simulink library "UAVdesign_net"  (Simulink 7.7)
settings: Solver=ode45  SolverMode=SingleTasking  StartTime=0.0  StopTime=10.0  RelTol=1e-3
undefined symbols (not defined in the file or in its folder): alpha_IERA_IELA_IELA, R_IERA_RA_RA
libraries: UAVdesign_net x75, simulink x13
(part 5 of 8)

== system UAVdesign_net/Utilities/Math/Quaternion Modulus ==
  q : Inport
  Math Function : Math  Operator=sqrt  SaturateOnIntegerOverflow=on
  Quaternion Norm : UAVdesign_net/Utilities/Math/Quaternion Norm  SystemSampleTime=-1
  |q| : Outport
  wires:
  Math Function/1 -> |q|/1
  q/1 -> Quaternion Norm/1
  Quaternion Norm/1 -> Math Function/1

== system UAVdesign_net/Utilities/Math/Quaternion Multiplication ==
  q : Inport
  r : Inport  Port=2
  Mux : Mux
  q0 : Subsystem
  q1 : Subsystem
  q2 : Subsystem
  q3 : Subsystem
  q*r : Outport
  wires:
  q/1 -> q0/1(q), q1/1(q), q2/1(q), q3/1(q)
  r/1 -> q0/2(r), q1/2(r), q2/2(r), q3/2(r)
  q0/1(q0) -> Mux/1
  q1/1(q1) -> Mux/2
  q2/1(q2) -> Mux/3
  q3/1(q3) -> Mux/4
  Mux/1 -> q*r/1

== system UAVdesign_net/Utilities/Math/Quaternion Norm ==
  q : Inport
  Demux : Demux
  Product{,1..3} (4 alike) : Product
  Sum : Sum  Inputs=4
  norm(q) : Outport
  wires:
  q/1 -> Demux/1
  Sum/1 -> norm(q)/1
  Product/1 -> Sum/1
  Product1/1 -> Sum/2
  Product2/1 -> Sum/3
  Product3/1 -> Sum/4
  Demux/1 -> Product/2, Product/1
  Demux/2 -> Product1/2, Product1/1
  Demux/3 -> Product2/2, Product2/1
  Demux/4 -> Product3/2, Product3/1

== system UAVdesign_net/Utilities/Math/Quaternion Normalize ==
  q : Inport
  Demux : Demux
  Mux : Mux
  Product{,1..3} (4 alike) : Product  Inputs=*/
  Quaternion Modulus : UAVdesign_net/Utilities/Math/Quaternion Modulus  SystemSampleTime=-1
  normal(q) : Outport
  wires:
  Demux/4 -> Product3/1
  Demux/3 -> Product2/1
  Demux/2 -> Product1/1
  Demux/1 -> Product/1
  Mux/1 -> normal(q)/1
  q/1 -> Quaternion Modulus/1, Demux/1
  Quaternion Modulus/1 -> Product1/2, Product/2, Product2/2, Product3/2
  Product/1 -> Mux/1
  Product1/1 -> Mux/2
  Product2/1 -> Mux/3
  Product3/1 -> Mux/4

== system UAVdesign_net/Utilities/Math/Quaternion Rotation (B<E) ==
  q : Inport
  v : Inport  Port=2
  Mux : Mux  Inputs=3
  Quaternion Normalize : UAVdesign_net/Utilities/Math/Quaternion Normalize  SystemSampleTime=-1
  V1 : Subsystem
  V2 : Subsystem
  V3 : Subsystem
  q*vq : Outport
  wires:
  Mux/1 -> q*vq/1
  V3/1(V3) -> Mux/3
  V2/1(V2) -> Mux/2
  V1/1(V1) -> Mux/1
  v/1 -> V3/2(vec), V2/2(vec), V1/2(vec)
  q/1 -> Quaternion Normalize/1
  Quaternion Normalize/1 -> V3/1(q), V2/1(q), V1/1(q)

== system UAVdesign_net/Utilities/Math/Quaternion Rotation (E<B) ==
  q : Inport
  v : Inport  Port=2
  Mux : Mux  Inputs=3
  Quaternion Conjugate : UAVdesign_net/Utilities/Math/Quaternion Conjugate  SystemSampleTime=-1
  Quaternion Normalize : UAVdesign_net/Utilities/Math/Quaternion Normalize  SystemSampleTime=-1
  V1 : Subsystem
  V2 : Subsystem
  V3 : Subsystem
  q*vq : Outport
  wires:
  Quaternion Conjugate/1 -> V1/1(q), V2/1(q), V3/1(q)
  Quaternion Normalize/1 -> Quaternion Conjugate/1
  q/1 -> Quaternion Normalize/1
  v/1 -> V1/2(vec), V2/2(vec), V3/2(vec)
  V1/1(V1) -> Mux/1
  V2/1(V2) -> Mux/2
  V3/1(V3) -> Mux/3
  Mux/1 -> q*vq/1

== system UAVdesign_net/Utilities/Math/Quaternion to Vector ==
  q : Inport
  Selector : Selector  InputPortWidth=4  IndexOptions=Index vector (dialog)  Indices=[2 3 4]  OutputSizes=1
  v : Outport
  wires:
  Selector/1 -> v/1
  q/1 -> Selector/1

== system UAVdesign_net/Utilities/Math/SinCos ==
  theta : Inport
  cosine : Trigonometry  Operator=cos
  sine : Trigonometry
  sin(theta) : Outport
  cos(theta) : Outport  Port=2
  wires:
  theta/1 -> sine/1, cosine/1
  sine/1 -> sin(theta)/1
  cosine/1 -> cos(theta)/1

== system UAVdesign_net/Utilities/Math/Transpose ==
  In : Inport
  Permute Dimensions : PermuteDimensions
  Out : Outport
  wires:
  In/1 -> Permute Dimensions/1
  Permute Dimensions/1 -> Out/1

== system UAVdesign_net/Utilities/Math/Vector to Quaternion ==
  v : Inport
  Ground : Ground
  Mux : Mux  Inputs=2
  q : Outport
  wires:
  Ground/1 -> Mux/1
  v/1 -> Mux/2
  Mux/1 -> q/1

== system UAVdesign_net/Utilities/Unit Conversion/Angle Conversion ==
  In1 : Inport
  Unit Conversion : Gain  Gain=slope  SaturateOnIntegerOverflow=on  OutDataTypeStr=Inherit: Same as input  ParamDataTypeStr=Inherit: Same as input
  Out1 : Outport
  wires:
  Unit Conversion/1 -> Out1/1
  In1/1 -> Unit Conversion/1

== system UAVdesign_net/Vehicle Models/Helicopter Model/6 DoF EoM ==
  Environment : Inport  OutDataTypeStr=Bus: Environment
  x : Inport  Port=2
  m : Inport  Port=3
  Inb : Inport  Port=4
  FM_MR : Inport  Port=5
  FM_TR : Inport  Port=6
  FM_FUSE : Inport  Port=7
  FM_HW : Inport  Port=8
  FM_VF : Inport  Port=9
  6DoF Equations of Motion : UAVdesign_net/Equations of Motion/6DoF Equations of Motion  SystemSampleTime=-1
  Add : Sum  Inputs=+++++
  Bus Selector1 : BusSelector  OutputSignals=g
  Constant : Constant  Value=[0 0]
  Constant1 : Constant  Value=[0 0 0 0]
  Constant2 : Constant  Value=[0 0 0 0]
  Constant3 : Constant  Value=[0 0 0]
  Demux : Demux  Outputs=2
  Demux1 : Demux  Outputs=[4 4 3 3 3 3]
  Mux : Mux  Inputs=2
  Mux2 : Mux  Inputs=2
  Product : Product  RndMeth=Zero
  Product1 : Product  Multiplication=Matrix(*)  RndMeth=Zero
  Rotation Matrix from Earth to Body : UAVdesign_net/Utilities/Axes/Euler Rotation Matrix from Earth to Body  SystemSampleTime=-1
  Sum : Sum  Inputs=++|
  Terminator : Terminator
  Terminator1 : Terminator
  Vector Concatenate1 : Concatenate  NumInputs=6  Mode=Vector
  Vector Concatenate6 : Concatenate  NumInputs=6  Mode=Vector
  x_dot : Outport
  FM_CG : Outport  Port=2  PortDimensions=36
  FM_Gravity : Outport  Port=3  PortDimensions=6
  wires:
  Mux2/1 -> FM_Gravity/1, Vector Concatenate6/1  "FM_CG"
  Vector Concatenate6/1 -> FM_CG/1
  Constant3/1 -> Mux2/2
  Vector Concatenate1/1 -> x_dot/1
  6DoF Equations of Motion/4 -> Vector Concatenate1/6  "alpha_E_dot"
  6DoF Equations of Motion/2 -> Vector Concatenate1/5  "omega_B_dot"
  6DoF Equations of Motion/3 -> Vector Concatenate1/4  "R_E_dot"
  6DoF Equations of Motion/1 -> Vector Concatenate1/3  "V_B_dot"
  Constant2/1 -> Vector Concatenate1/2  "p_BE_ddot"
  Constant1/1 -> Vector Concatenate1/1  "p_BE_dot"
  Demux1/1 -> Terminator1/1  "p_BE"
  Demux1/2 -> Terminator/1  "p_BE_dot"
  Demux1/4 -> 6DoF Equations of Motion/3  "R_E"
  Demux1/5 -> 6DoF Equations of Motion/2  "omega_B"
  Demux1/3 -> 6DoF Equations of Motion/1  "V_B"
  Demux1/6 -> Rotation Matrix from Earth to Body/1, 6DoF Equations of Motion/4  "alpha_E"
  Add/1 -> Demux/1
  FM_VF/1 -> Vector Concatenate6/6, Add/5  "FM_VF"
  FM_HW/1 -> Vector Concatenate6/5, Add/4  "FM_HW"
  FM_FUSE/1 -> Vector Concatenate6/4, Add/3  "FM_FUSE"
  FM_TR/1 -> Vector Concatenate6/3, Add/2  "FM_TR"
  FM_MR/1 -> Vector Concatenate6/2, Add/1  "FM_MR"
  Mux/1 -> Product1/2
  Product1/1 -> Mux2/1, Sum/1
  Sum/1 -> 6DoF Equations of Motion/5
  Demux/1 -> Sum/2  "F"
  Rotation Matrix from Earth to Body/1 -> Product1/1
  Product/1 -> Mux/2
  Constant/1 -> Mux/1
  Bus Selector1/1 -> Product/1  "<g>"
  Environment/1 -> Bus Selector1/1
  x/1 -> Demux1/1
  Inb/1 -> 6DoF Equations of Motion/8
  m/1 -> Product/2, 6DoF Equations of Motion/7
  Demux/2 -> 6DoF Equations of Motion/6  "M"

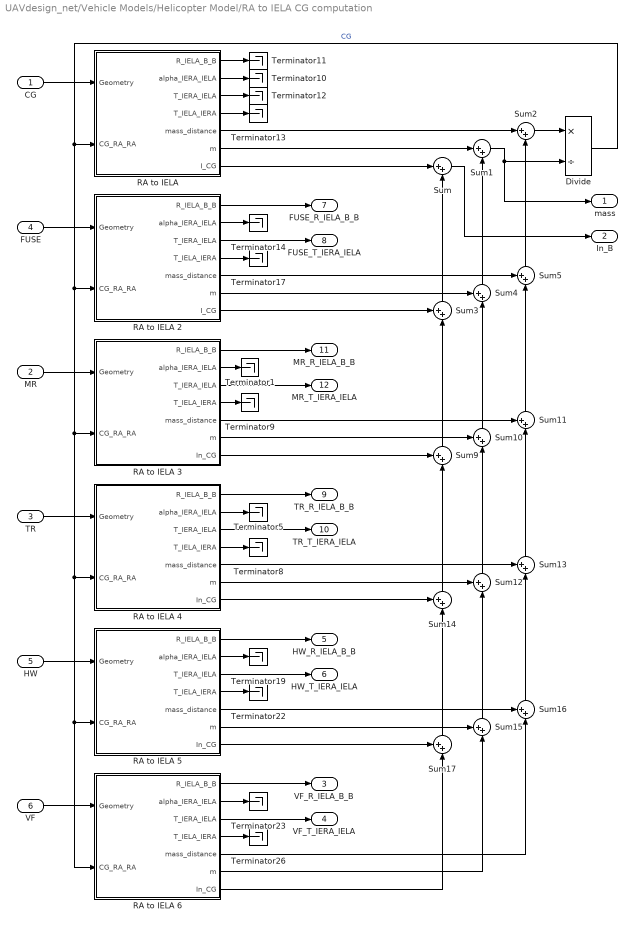
== system UAVdesign_net/Vehicle Models/Helicopter Model/RA to IELA CG computation ==
  CG : Inport  OutDataTypeStr=Bus: GeometryParameters
  MR : Inport  Port=2  OutDataTypeStr=Bus: GeometryParameters
  TR : Inport  Port=3  OutDataTypeStr=Bus: GeometryParameters
  FUSE : Inport  Port=4  OutDataTypeStr=Bus: GeometryParameters
  HW : Inport  Port=5  OutDataTypeStr=Bus: GeometryParameters
  VF : Inport  Port=6  OutDataTypeStr=Bus: GeometryParameters
  Divide : Product  Inputs=*/
  RA to IELA : Subsystem
      mask Display:
      | port_label('input', 1, 'Geometry', 'texmode', 'on')
      | port_label('input', 2, 'R_{CG-RA|RA}', 'texmode', 'on')
      | port_label('output', 1, 'R_{IELA-B|B}', 'texmode', 'on')
      | port_label('output', 2, '\alpha_{IERA-IELA|IELA}', 'texmode', 'on')
      | port_label('output', 3, 'T_{IERA-IELA}', 'texmode', 'on')
      | port_label('output', 4, 'T_{IELA-IERA}', 'texmode', 'on')
      | port_label('output', 5, 'mass x distance', 'texmode', 'on')
      | port_label('output', 6, 'mass', 'texmode', 'on')
      | port_label('output', 7, 'I_{B}', 'texmode', 'on')
  RA to IELA 2 : Subsystem
      mask Display:
      | port_label('input', 1, 'Geometry', 'texmode', 'on')
      | port_label('input', 2, 'R_{CG-RA|RA}', 'texmode', 'on')
      | port_label('output', 1, 'R_{IELA-B|B}', 'texmode', 'on')
      | port_label('output', 2, '\alpha_{IERA-IELA|IELA}', 'texmode', 'on')
      | port_label('output', 3, 'T_{IERA-IELA}', 'texmode', 'on')
      | port_label('output', 4, 'T_{IELA-IERA}', 'texmode', 'on')
      | port_label('output', 5, 'mass x distance', 'texmode', 'on')
      | port_label('output', 6, 'mass', 'texmode', 'on')
      | port_label('output', 7, 'I_{B}', 'texmode', 'on')
  RA to IELA 3 : Subsystem
      mask Display:
      | port_label('input', 1, 'Geometry', 'texmode', 'on')
      | port_label('input', 2, 'R_{CG-RA|RA}', 'texmode', 'on')
      | port_label('output', 1, 'R_{IELA-B|B}', 'texmode', 'on')
      | port_label('output', 2, '\alpha_{IERA-IELA|IELA}', 'texmode', 'on')
      | port_label('output', 3, 'T_{IERA-IELA}', 'texmode', 'on')
      | port_label('output', 4, 'T_{IELA-IERA}', 'texmode', 'on')
      | port_label('output', 5, 'mass x distance', 'texmode', 'on')
      | port_label('output', 6, 'mass', 'texmode', 'on')
      | port_label('output', 7, 'In_{B}', 'texmode', 'on')
  RA to IELA 4 : Subsystem
      mask Display:
      | port_label('input', 1, 'Geometry', 'texmode', 'on')
      | port_label('input', 2, 'R_{CG-RA|RA}', 'texmode', 'on')
      | port_label('output', 1, 'R_{IELA-B|B}', 'texmode', 'on')
      | port_label('output', 2, '\alpha_{IERA-IELA|IELA}', 'texmode', 'on')
      | port_label('output', 3, 'T_{IERA-IELA}', 'texmode', 'on')
      | port_label('output', 4, 'T_{IELA-IERA}', 'texmode', 'on')
      | port_label('output', 5, 'mass x distance', 'texmode', 'on')
      | port_label('output', 6, 'mass', 'texmode', 'on')
      | port_label('output', 7, 'In_{B}', 'texmode', 'on')
  RA to IELA 5 : Subsystem
      mask Display:
      | port_label('input', 1, 'Geometry', 'texmode', 'on')
      | port_label('input', 2, 'R_{CG-RA|RA}', 'texmode', 'on')
      | port_label('output', 1, 'R_{IELA-B|B}', 'texmode', 'on')
      | port_label('output', 2, '\alpha_{IERA-IELA|IELA}', 'texmode', 'on')
      | port_label('output', 3, 'T_{IERA-IELA}', 'texmode', 'on')
      | port_label('output', 4, 'T_{IELA-IERA}', 'texmode', 'on')
      | port_label('output', 5, 'mass x distance', 'texmode', 'on')
      | port_label('output', 6, 'mass', 'texmode', 'on')
      | port_label('output', 7, 'In_{B}', 'texmode', 'on')
  RA to IELA 6 : Subsystem
      mask Display:
      | port_label('input', 1, 'Geometry', 'texmode', 'on')
      | port_label('input', 2, 'R_{CG-RA|RA}', 'texmode', 'on')
      | port_label('output', 1, 'R_{IELA-B|B}', 'texmode', 'on')
      | port_label('output', 2, '\alpha_{IERA-IELA|IELA}', 'texmode', 'on')
      | port_label('output', 3, 'T_{IERA-IELA}', 'texmode', 'on')
      | port_label('output', 4, 'T_{IELA-IERA}', 'texmode', 'on')
      | port_label('output', 5, 'mass x distance', 'texmode', 'on')
      | port_label('output', 6, 'mass', 'texmode', 'on')
      | port_label('output', 7, 'In_{B}', 'texmode', 'on')
  Sum : Sum  Inputs=|++
  Sum1 : Sum  Inputs=|++
  Sum{3..5,9..17} (12 alike) : Sum  Inputs=++|
  Sum2 : Sum  Inputs=|++
  Terminator{1,5,8..14,17,19,22..23,26} (14 alike) : Terminator
  mass : Outport
  In_B : Outport  Port=2
  VF_R_IELA_B_B : Outport  Port=3
  VF_T_IERA_IELA : Outport  Port=4
  HW_R_IELA_B_B : Outport  Port=5
  HW_T_IERA_IELA : Outport  Port=6
  FUSE_R_IELA_B_B : Outport  Port=7
  FUSE_T_IERA_IELA : Outport  Port=8
  TR_R_IELA_B_B : Outport  Port=9
  TR_T_IERA_IELA : Outport  Port=10
  MR_R_IELA_B_B : Outport  Port=11
  MR_T_IERA_IELA : Outport  Port=12
  wires:
  RA to IELA 6/3(T_IERA_IELA) -> VF_T_IERA_IELA/1
  RA to IELA 6/1(R_IELA_B_B) -> VF_R_IELA_B_B/1
  RA to IELA 5/3(T_IERA_IELA) -> HW_T_IERA_IELA/1
  RA to IELA 5/1(R_IELA_B_B) -> HW_R_IELA_B_B/1
  RA to IELA 4/3(T_IERA_IELA) -> TR_T_IERA_IELA/1
  RA to IELA 4/1(R_IELA_B_B) -> TR_R_IELA_B_B/1
  RA to IELA 2/3(T_IERA_IELA) -> FUSE_T_IERA_IELA/1
  RA to IELA 2/1(R_IELA_B_B) -> FUSE_R_IELA_B_B/1
  RA to IELA 6/6(m) -> Sum15/2
  RA to IELA 6/5(mass_distance) -> Sum16/2
  RA to IELA 6/7(In_CG) -> Sum17/2
  RA to IELA 6/4(T_IELA_IERA) -> Terminator26/1
  RA to IELA 6/2(alpha_IERA_IELA) -> Terminator23/1
  VF/1 -> RA to IELA 6/1(Geometry)
  RA to IELA 5/6(m) -> Sum15/1
  RA to IELA 5/5(mass_distance) -> Sum16/1
  Sum16/1 -> Sum13/2
  Sum15/1 -> Sum12/2
  Sum17/1 -> Sum14/2
  RA to IELA 5/7(In_CG) -> Sum17/1
  RA to IELA 5/4(T_IELA_IERA) -> Terminator22/1
  RA to IELA 5/2(alpha_IERA_IELA) -> Terminator19/1
  HW/1 -> RA to IELA 5/1(Geometry)
  RA to IELA 4/6(m) -> Sum12/1
  RA to IELA 4/5(mass_distance) -> Sum13/1
  Sum13/1 -> Sum11/2
  Sum12/1 -> Sum10/2
  Sum14/1 -> Sum9/2
  RA to IELA 4/7(In_CG) -> Sum14/1
  RA to IELA 3/5(mass_distance) -> Sum11/1
  RA to IELA 3/6(m) -> Sum10/1
  Sum11/1 -> Sum5/2
  Sum10/1 -> Sum4/2
  Sum9/1 -> Sum3/2
  RA to IELA 3/7(In_CG) -> Sum9/1
  FUSE/1 -> RA to IELA 2/1(Geometry)
  Sum2/1 -> Divide/1
  Sum1/1 -> mass/1, Divide/2
  Sum/1 -> In_B/1
  Sum5/1 -> Sum2/2
  Sum4/1 -> Sum1/2
  Sum3/1 -> Sum/2
  RA to IELA 2/7(I_CG) -> Sum3/1
  RA to IELA 2/5(mass_distance) -> Sum5/1
  RA to IELA 2/6(m) -> Sum4/1
  RA to IELA 2/4(T_IELA_IERA) -> Terminator17/1
  RA to IELA 2/2(alpha_IERA_IELA) -> Terminator14/1
  RA to IELA/5(mass_distance) -> Sum2/1
  RA to IELA/6(m) -> Sum1/1
  RA to IELA/7(I_CG) -> Sum/1
  RA to IELA/4(T_IELA_IERA) -> Terminator13/1
  RA to IELA/3(T_IERA_IELA) -> Terminator12/1
  RA to IELA/1(R_IELA_B_B) -> Terminator11/1
  RA to IELA/2(alpha_IERA_IELA) -> Terminator10/1
  CG/1 -> RA to IELA/1(Geometry)
  Divide/1 -> RA to IELA 3/2(CG_RA_RA), RA to IELA 4/2(CG_RA_RA), RA to IELA 5/2(CG_RA_RA), RA to IELA 6/2(CG_RA_RA), RA to IELA 2/2(CG_RA_RA), RA to IELA/2(CG_RA_RA)  "CG"
  RA to IELA 3/4(T_IELA_IERA) -> Terminator9/1
  RA to IELA 4/4(T_IELA_IERA) -> Terminator8/1
  RA to IELA 4/2(alpha_IERA_IELA) -> Terminator5/1
  TR/1 -> RA to IELA 4/1(Geometry)
  RA to IELA 3/3(T_IERA_IELA) -> MR_T_IERA_IELA/1
  RA to IELA 3/2(alpha_IERA_IELA) -> Terminator1/1
  RA to IELA 3/1(R_IELA_B_B) -> MR_R_IELA_B_B/1
  MR/1 -> RA to IELA 3/1(Geometry)

== system UAVdesign_net/Vehicle Models/Helicopter Model/Wash Coupling ==
  d_vector : Inport
  ParametersBus : Inport  Port=2
  GeometryBus : Inport  Port=3
  Bus Selector : BusSelector  OutputSignals=MR.radius
  Bus Selector1 : BusSelector  OutputSignals=MR.R_IERA_RA_RA,TR.R_IERA_RA_RA,FUSE.R_IERA_RA_RA,HW.R_IERA_RA_RA,VF.R_IERA_RA_RA
  Vector Concatenate1 : Concatenate  NumInputs=5  Mode=Vector
  Wash Coupling : Stateflow chart  TreatAsAtomicUnit=on
  V_W_omega_W_vector : Outport
  wires:
  Bus Selector1/5 -> Vector Concatenate1/5  "<R_IERA_RA_RA>"
  Bus Selector1/4 -> Vector Concatenate1/4  "<R_IERA_RA_RA>"
  Bus Selector1/3 -> Vector Concatenate1/3  "<R_IERA_RA_RA>"
  Bus Selector1/2 -> Vector Concatenate1/2  "<R_IERA_RA_RA>"
  Bus Selector1/1 -> Vector Concatenate1/1  "<R_IERA_RA_RA>"
  Vector Concatenate1/1 -> Wash Coupling/2(R)
  GeometryBus/1 -> Bus Selector1/1
  Bus Selector/1 -> Wash Coupling/3(MR_radius)  "<radius>"
  ParametersBus/1 -> Bus Selector/1
  Wash Coupling/1(vw_omw) -> V_W_omega_W_vector/1
  d_vector/1 -> Wash Coupling/1(d)

== system UAVdesign_net/Vehicle Models/Helicopter Parameters/Fin Parameters ==
  In : Inport
  Bus Creator : BusCreator  Inputs=14  OutDataTypeStr=Bus: FinParameters  NonVirtualBus=on
  Demux : Demux  Outputs=14
  Gain{,1..3} (4 alike) : Gain  Gain=pi/180
  Parameters : Outport  OutDataTypeStr=Bus: FinParameters
  wires:
  In/1 -> Demux/1
  Bus Creator/1 -> Parameters/1
  Demux/1 -> Bus Creator/1  "span"
  Demux/2 -> Bus Creator/2  "chord"
  Demux/3 -> Gain2/1
  Gain2/1 -> Bus Creator/3  "dihedral"
  Demux/4 -> Gain/1
  Gain/1 -> Bus Creator/4  "incid"
  Gain1/1 -> Bus Creator/5  "sweep"
  Demux/5 -> Gain1/1
  Demux/6 -> Bus Creator/6  "taper"
  Demux/7 -> Gain3/1
  Gain3/1 -> Bus Creator/7  "stall"
  Demux/8 -> Bus Creator/8  "a0"
  Demux/9 -> Bus Creator/9  "a1s2"
  Demux/10 -> Bus Creator/10  "cd0"
  Demux/11 -> Bus Creator/11  "cd1s1"
  Demux/12 -> Bus Creator/12  "cd2c1"
  Demux/13 -> Bus Creator/13  "cm0"
  Demux/14 -> Bus Creator/14  "cm1s1"

== system UAVdesign_net/Vehicle Models/Helicopter Parameters/Fin Parameters1 ==
  In : Inport
  Bus Creator : BusCreator  Inputs=14  OutDataTypeStr=Bus: FinParameters  NonVirtualBus=on
  Demux : Demux  Outputs=14
  Gain{,1..3} (4 alike) : Gain  Gain=pi/180
  Parameters : Outport  OutDataTypeStr=Bus: FinParameters
  wires:
  Demux/14 -> Bus Creator/14  "cm1s1"
  Demux/13 -> Bus Creator/13  "cm0"
  Demux/12 -> Bus Creator/12  "cd2c1"
  Demux/11 -> Bus Creator/11  "cd1s1"
  Demux/10 -> Bus Creator/10  "cd0"
  Demux/9 -> Bus Creator/9  "a1s2"
  Demux/8 -> Bus Creator/8  "a0"
  Gain3/1 -> Bus Creator/7  "stall"
  Demux/7 -> Gain3/1
  Demux/6 -> Bus Creator/6  "taper"
  Demux/5 -> Gain1/1
  Gain1/1 -> Bus Creator/5  "sweep"
  Gain/1 -> Bus Creator/4  "incid"
  Demux/4 -> Gain/1
  Gain2/1 -> Bus Creator/3  "dihedral"
  Demux/3 -> Gain2/1
  Demux/2 -> Bus Creator/2  "chord"
  Demux/1 -> Bus Creator/1  "span"
  Bus Creator/1 -> Parameters/1
  In/1 -> Demux/1

== system UAVdesign_net/Vehicle Models/Helicopter Parameters/Fuse Parameters ==
  In : Inport
  Bus Creator : BusCreator  Inputs=7  OutDataTypeStr=Bus: FuselageParameters  NonVirtualBus=on
  Demux : Demux  Outputs=17
  Vector Concatenate{,1..4} (5 alike) : Concatenate  NumInputs=3  Mode=Vector
  Parameters : Outport  OutDataTypeStr=Bus: FuselageParameters
  wires:
  Demux/1 -> Bus Creator/1  "carea"
  Bus Creator/1 -> Parameters/1
  In/1 -> Demux/1
  Demux/2 -> Bus Creator/2  "clen"
  Demux/3 -> Vector Concatenate/1
  Demux/4 -> Vector Concatenate/2
  Demux/5 -> Vector Concatenate/3
  Vector Concatenate/1 -> Bus Creator/3  "cx"
  Demux/6 -> Vector Concatenate1/1
  Demux/7 -> Vector Concatenate1/2
  Demux/8 -> Vector Concatenate1/3
  Vector Concatenate1/1 -> Bus Creator/4  "cy"
  Demux/9 -> Vector Concatenate2/1
  Demux/10 -> Vector Concatenate2/2
  Demux/11 -> Vector Concatenate2/3
  Vector Concatenate2/1 -> Bus Creator/5  "cz"
  Demux/12 -> Vector Concatenate3/1
  Demux/13 -> Vector Concatenate3/2
  Demux/14 -> Vector Concatenate3/3
  Demux/15 -> Vector Concatenate4/1
  Demux/16 -> Vector Concatenate4/2
  Demux/17 -> Vector Concatenate4/3
  Vector Concatenate3/1 -> Bus Creator/6  "cm"
  Vector Concatenate4/1 -> Bus Creator/7  "cn"

== system UAVdesign_net/Vehicle Models/Helicopter Parameters/Rotor Parameters ==
  In : Inport
  Bus Creator : BusCreator  Inputs=18  OutDataTypeStr=Bus: RotorParameters  NonVirtualBus=on
  Data Type Conversion : DataTypeConversion  OutDataTypeStr=int32  RndMeth=Nearest
  Data Type Conversion1 : DataTypeConversion  OutDataTypeStr=uint32  RndMeth=Nearest
  Demux : Demux  Outputs=20
  Gain : Gain  Gain=pi/180
  Gain1 : Gain  Gain=pi/180
  Gain2 : Gain  Gain=180/pi
  Gain3 : Gain  Gain=pi/180
  Vector Concatenate : Concatenate  NumInputs=3  Mode=Vector
  Parameters : Outport  OutDataTypeStr=Bus: RotorParameters
  wires:
  Demux/20 -> Bus Creator/18  "azsign"
  Demux/18 -> Bus Creator/16  "lmast"
  Demux/17 -> Bus Creator/15  "mbar"
  Demux/16 -> Bus Creator/14  "iflap"
  Demux/13 -> Bus Creator/11  "btmax"
  Demux/1 -> Bus Creator/1  "a0"
  Bus Creator/1 -> Parameters/1
  Demux/4 -> Vector Concatenate/3
  Demux/3 -> Vector Concatenate/2
  Demux/2 -> Vector Concatenate/1
  Vector Concatenate/1 -> Bus Creator/2  "del0_2"
  In/1 -> Demux/1
  Data Type Conversion/1 -> Bus Creator/17  "hubtype"
  Demux/19 -> Data Type Conversion/1
  Gain/1 -> Bus Creator/3  "precone"
  Gain1/1 -> Bus Creator/4  "delta3"
  Gain2/1 -> Bus Creator/6  "khub"
  Gain3/1 -> Bus Creator/13  "twist"
  Demux/5 -> Gain/1
  Demux/6 -> Gain1/1
  Demux/7 -> Bus Creator/5  "e"
  Demux/8 -> Gain2/1
  Data Type Conversion1/1 -> Bus Creator/7  "nb"
  Demux/9 -> Data Type Conversion1/1
  Demux/10 -> Bus Creator/8  "radius"
  Demux/11 -> Bus Creator/9  "chord"
  Demux/12 -> Bus Creator/10  "btmin"
  Demux/15 -> Gain3/1
  Demux/14 -> Bus Creator/12  "btq"

== system UAVdesign_net/Vehicle Models/Helicopter Parameters/Rotor Parameters1 ==
  In : Inport
  Bus Creator : BusCreator  Inputs=18  OutDataTypeStr=Bus: RotorParameters  NonVirtualBus=on
  Data Type Conversion : DataTypeConversion  OutDataTypeStr=int32  RndMeth=Nearest
  Data Type Conversion1 : DataTypeConversion  OutDataTypeStr=uint32  RndMeth=Nearest
  Demux : Demux  Outputs=20
  Gain : Gain  Gain=pi/180
  Gain1 : Gain  Gain=pi/180
  Gain2 : Gain  Gain=180/pi
  Gain3 : Gain  Gain=pi/180
  Vector Concatenate : Concatenate  NumInputs=3  Mode=Vector
  Parameters : Outport  OutDataTypeStr=Bus: RotorParameters
  wires:
  Demux/14 -> Bus Creator/12  "btq"
  Demux/15 -> Gain3/1
  Demux/12 -> Bus Creator/10  "btmin"
  Demux/11 -> Bus Creator/9  "chord"
  Demux/10 -> Bus Creator/8  "radius"
  Demux/9 -> Data Type Conversion1/1
  Data Type Conversion1/1 -> Bus Creator/7  "nb"
  Demux/8 -> Gain2/1
  Demux/7 -> Bus Creator/5  "e"
  Demux/6 -> Gain1/1
  Demux/5 -> Gain/1
  Gain3/1 -> Bus Creator/13  "twist"
  Gain2/1 -> Bus Creator/6  "khub"
  Gain1/1 -> Bus Creator/4  "delta3"
  Gain/1 -> Bus Creator/3  "precone"
  Demux/19 -> Data Type Conversion/1
  Data Type Conversion/1 -> Bus Creator/17  "hubtype"
  In/1 -> Demux/1
  Vector Concatenate/1 -> Bus Creator/2  "del0_2"
  Demux/2 -> Vector Concatenate/1
  Demux/3 -> Vector Concatenate/2
  Demux/4 -> Vector Concatenate/3
  Bus Creator/1 -> Parameters/1
  Demux/1 -> Bus Creator/1  "a0"
  Demux/13 -> Bus Creator/11  "btmax"
  Demux/16 -> Bus Creator/14  "iflap"
  Demux/17 -> Bus Creator/15  "mbar"
  Demux/18 -> Bus Creator/16  "lmast"
  Demux/20 -> Bus Creator/18  "azsign"

== system UAVdesign_net/Vehicle Models/Quad-Rotor Model (Momentum)/6 DoF EoM ==
  Environment : Inport
  x : Inport  Port=2
  m : Inport  Port=3
  Inb : Inport  Port=4
  FM_ROT : Inport  Port=5
  FM_FUSE : Inport  Port=6
  6DoF Equations of Motion (Quaternions) : UAVdesign_net/Equations of Motion/6DoF Equations of Motion (Quaternions)  SystemSampleTime=-1
  Add : Sum  Inputs=+++++
  Bus Selector1 : BusSelector  OutputSignals=g
  Constant : Constant  Value=[0 0]
  Constant3 : Constant  Value=[0 0 0]
  Demux : Demux  Outputs=2
  Demux1 : Demux  Outputs=[3 3 3 4]
  Demux2 : Demux
  Mux : Mux  Inputs=2
  Mux2 : Mux  Inputs=2
  Product : Product  RndMeth=Zero
  Quaternion Rotation (B<E) : UAVdesign_net/Utilities/Math/Quaternion Rotation (B<E)  SystemSampleTime=-1
  Sum : Sum  Inputs=++|
  Vector Concatenate1 : Concatenate  NumInputs=4  Mode=Vector
  Vector Concatenate6 : Concatenate  NumInputs=3  Mode=Vector
  x_dot : Outport
  FM_CG : Outport  Port=2  PortDimensions=36
  FM_Gravity : Outport  Port=3  PortDimensions=6
  wires:
  Demux/2 -> 6DoF Equations of Motion (Quaternions)/6  "M"
  m/1 -> Product/2, 6DoF Equations of Motion (Quaternions)/7
  Inb/1 -> 6DoF Equations of Motion (Quaternions)/8
  x/1 -> Demux1/1
  Environment/1 -> Bus Selector1/1
  Bus Selector1/1 -> Product/1  "<g>"
  Constant/1 -> Mux/1
  Product/1 -> Mux/2
  Demux/1 -> Sum/2  "F"
  Sum/1 -> 6DoF Equations of Motion (Quaternions)/5
  Add/1 -> Demux/1
  Vector Concatenate1/1 -> x_dot/1
  Constant3/1 -> Mux2/2
  Vector Concatenate6/1 -> FM_CG/1
  FM_FUSE/1 -> Vector Concatenate6/3, Add/5  "FM_FUSE"
  FM_ROT/1 -> Vector Concatenate6/2, Demux2/1  "FM_ROT"
  Mux2/1 -> Vector Concatenate6/1, FM_Gravity/1  "FM_CG"
  Mux/1 -> Quaternion Rotation (B<E)/2
  Demux1/1 -> 6DoF Equations of Motion (Quaternions)/1
  Demux1/2 -> 6DoF Equations of Motion (Quaternions)/2
  Demux1/3 -> 6DoF Equations of Motion (Quaternions)/3
  Demux1/4 -> 6DoF Equations of Motion (Quaternions)/4, Quaternion Rotation (B<E)/1
  Quaternion Rotation (B<E)/1 -> Sum/1, Mux2/1
  6DoF Equations of Motion (Quaternions)/1 -> Vector Concatenate1/1
  6DoF Equations of Motion (Quaternions)/2 -> Vector Concatenate1/2
  6DoF Equations of Motion (Quaternions)/3 -> Vector Concatenate1/3
  6DoF Equations of Motion (Quaternions)/4 -> Vector Concatenate1/4
  Demux2/1 -> Add/1
  Demux2/2 -> Add/2
  Demux2/3 -> Add/3
  Demux2/4 -> Add/4

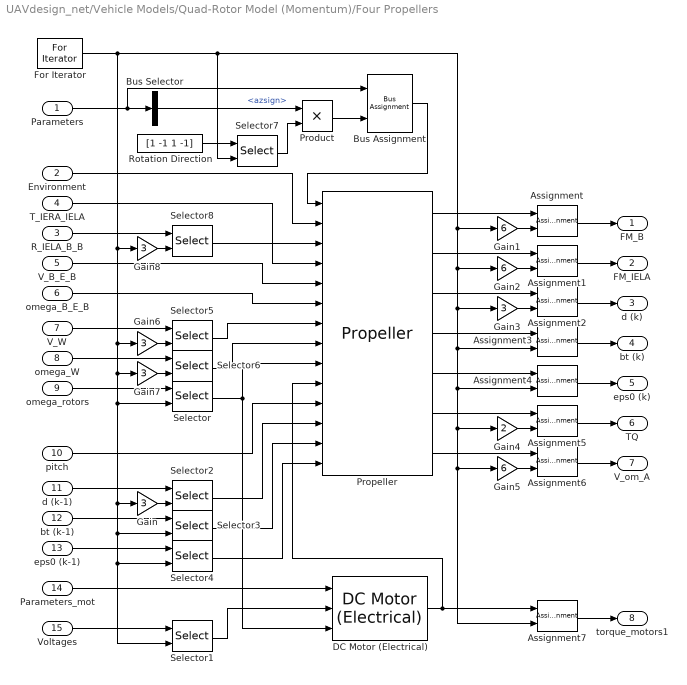
== system UAVdesign_net/Vehicle Models/Quad-Rotor Model (Momentum)/Four Propellers ==
  Parameters : Inport
  Environment : Inport  Port=2
  R_IELA_B_B : Inport  Port=3  PortDimensions=12
  T_IERA_IELA : Inport  Port=4  PortDimensions=[3 3]
  V_B_E_B : Inport  Port=5  PortDimensions=3
  omega_B_E_B : Inport  Port=6  PortDimensions=3
  V_W : Inport  Port=7  PortDimensions=12
  omega_W : Inport  Port=8  PortDimensions=12
  omega_rotors : Inport  Port=9  PortDimensions=4
  pitch : Inport  Port=10  PortDimensions=1
  d (k-1) : Inport  Port=11  PortDimensions=12
  bt (k-1) : Inport  Port=12  PortDimensions=4
  eps0 (k-1) : Inport  Port=13  PortDimensions=4
  Parameters_mot : Inport  Port=14
  Voltages : Inport  Port=15  PortDimensions=4
  Assignment : Assignment  IndexMode=Zero-based  OutputInitialize=Specify size for each dimension in table  IndexOptions=Starting index (port)  Indices=1  OutputSizes=24
  Assignment1 : Assignment  IndexMode=Zero-based  OutputInitialize=Specify size for each dimension in table  IndexOptions=Starting index (port)  Indices=1  OutputSizes=24
  Assignment2 : Assignment  IndexMode=Zero-based  OutputInitialize=Specify size for each dimension in table  IndexOptions=Starting index (port)  Indices=1  OutputSizes=12
  Assignment3 : Assignment  IndexMode=Zero-based  OutputInitialize=Specify size for each dimension in table  IndexOptions=Starting index (port)  Indices=1  OutputSizes=4
  Assignment4 : Assignment  IndexMode=Zero-based  OutputInitialize=Specify size for each dimension in table  IndexOptions=Starting index (port)  Indices=1  OutputSizes=4
  Assignment5 : Assignment  IndexMode=Zero-based  OutputInitialize=Specify size for each dimension in table  IndexOptions=Starting index (port)  Indices=1  OutputSizes=8
  Assignment6 : Assignment  IndexMode=Zero-based  OutputInitialize=Specify size for each dimension in table  IndexOptions=Starting index (port)  Indices=1  OutputSizes=24
  Assignment7 : Assignment  IndexMode=Zero-based  OutputInitialize=Specify size for each dimension in table  IndexOptions=Starting index (port)  Indices=1  OutputSizes=4
  Bus Selector : BusSelector  OutputSignals=azsign
  Bus Assignment : BusAssignment  AssignedSignals=azsign
  DC Motor (Electrical) : UAVdesign_net/Subsystem Models/DC Motor (Electrical)  SystemSampleTime=-1
  For Iterator : ForIterator  ResetStates=reset  IterationLimit=4  IndexMode=Zero-based
  Gain{,3,6..8} (5 alike) : Gain  Gain=3  OutDataTypeStr=uint32
  Gain1 : Gain  Gain=6  OutDataTypeStr=uint32
  Gain2 : Gain  Gain=6  OutDataTypeStr=uint32
  Gain4 : Gain  Gain=2  OutDataTypeStr=uint32
  Gain5 : Gain  Gain=6  OutDataTypeStr=uint32
  Product : Product  RndMeth=Zero
  Propeller : UAVdesign_net/Subsystem Models/Propeller  SystemSampleTime=-1
  Rotation Direction : Constant  Value=[1 -1 1 -1]
  Selector{,1,3..4,7} (5 alike) : Selector  IndexMode=Zero-based  InputPortWidth=4  IndexOptions=Starting index (port)  Indices=[1 3]  OutputSizes=1
  Selector{2,5..6,8} (4 alike) : Selector  IndexMode=Zero-based  InputPortWidth=12  IndexOptions=Starting index (port)  Indices=[1 3]  OutputSizes=3
  FM_B : Outport
  FM_IELA : Outport  Port=2
  d (k) : Outport  Port=3
  bt (k) : Outport  Port=4
  eps0 (k) : Outport  Port=5
  TQ : Outport  Port=6
  V_om_A : Outport  Port=7
  torque_motors1 : Outport  Port=8
  wires:
  Voltages/1 -> Selector1/1
  Selector1/1 -> DC Motor (Electrical)/2
  Assignment7/1 -> torque_motors1/1
  DC Motor (Electrical)/1 -> Propeller/10, Assignment7/1
  Parameters_mot/1 -> DC Motor (Electrical)/1
  Selector4/1 -> Propeller/14
  Selector3/1 -> Propeller/13
  Selector2/1 -> Propeller/12
  pitch/1 -> Propeller/11
  Selector/1 -> DC Motor (Electrical)/3, Propeller/9
  Selector6/1 -> Propeller/8
  Selector5/1 -> Propeller/7
  Gain8/1 -> Selector8/2
  R_IELA_B_B/1 -> Selector8/1
  Selector8/1 -> Propeller/3
  Rotation Direction/1 -> Selector7/1
  Selector7/1 -> Product/2
  Product/1 -> Bus Assignment/2
  Bus Selector/1 -> Product/1  "<azsign>"
  Parameters/1 -> Bus Selector/1, Bus Assignment/1
  Bus Assignment/1 -> Propeller/1
  Gain7/1 -> Selector6/2
  Gain6/1 -> Selector5/2
  omega_W/1 -> Selector6/1
  V_W/1 -> Selector5/1
  Assignment6/1 -> V_om_A/1
  Propeller/7 -> Assignment6/1
  Gain5/1 -> Assignment6/2
  Assignment5/1 -> TQ/1
  Assignment4/1 -> eps0 (k)/1
  Assignment3/1 -> bt (k)/1
  Propeller/6 -> Assignment5/1
  Gain4/1 -> Assignment5/2
  Propeller/5 -> Assignment4/1
  Propeller/4 -> Assignment3/1
  Assignment2/1 -> d (k)/1
  Propeller/3 -> Assignment2/1
  Gain3/1 -> Assignment2/2
  Assignment1/1 -> FM_IELA/1
  Propeller/2 -> Assignment1/1
  Gain2/1 -> Assignment1/2
  Propeller/1 -> Assignment/1
  Gain1/1 -> Assignment/2
  Assignment/1 -> FM_B/1
  eps0 (k-1)/1 -> Selector4/1
  bt (k-1)/1 -> Selector3/1
  d (k-1)/1 -> Selector2/1
  Gain/1 -> Selector2/2
  For Iterator/1 -> Gain8/1, Gain6/1, Gain7/1, Gain/1, Selector1/2, Selector4/2, Selector3/2, Selector/2, Selector7/2, Assignment7/2, Gain5/1, Gain4/1, Assignment4/2, Assignment3/2, Gain3/1, Gain2/1, Gain1/1
  omega_rotors/1 -> Selector/1
  omega_B_E_B/1 -> Propeller/6
  V_B_E_B/1 -> Propeller/5
  T_IERA_IELA/1 -> Propeller/4
  Environment/1 -> Propeller/2

== system UAVdesign_net/Vehicle Models/Quad-Rotor Model (Momentum)/Four Propellers Rotation Dynamics ==
  Parameters : Inport
  torque_prop : Inport  Port=2  PortDimensions=4
  torque_mot : Inport  Port=3  PortDimensions=4
  omega_B_E_B : Inport  Port=4  PortDimensions=3
  omega_dot_B_E_B : Inport  Port=5  PortDimensions=3
  omega_rotors : Inport  Port=6  PortDimensions=4
  Assignment1 : Assignment  IndexMode=Zero-based  OutputInitialize=Specify size for each dimension in table  IndexOptions=Starting index (port)  Indices=1  OutputSizes=4
  Bus Selector : BusSelector  OutputSignals=azsign
  Bus Assignment : BusAssignment  AssignedSignals=azsign
  For Iterator : ForIterator  ResetStates=reset  IterationLimit=4  IndexMode=Zero-based
  Orientation : Constant  Value=eye(3,3)
  Product : Product  RndMeth=Zero
  Propeller Rotation Dynamics : UAVdesign_net/Subsystem Models/Propeller Rotation Dynamics  SystemSampleTime=-1
  Rotation Direction : Constant  Value=[1 -1 1 -1]
  Selector{1..3,7} (4 alike) : Selector  IndexMode=Zero-based  InputPortWidth=4  IndexOptions=Starting index (port)  Indices=[1 3]  OutputSizes=1
  omega_dot_motors : Outport
  wires:
  torque_mot/1 -> Selector3/1
  Selector3/1 -> Propeller Rotation Dynamics/4
  omega_rotors/1 -> Selector2/1
  Rotation Direction/1 -> Selector7/1
  Selector7/1 -> Product/2
  Product/1 -> Bus Assignment/2
  Bus Selector/1 -> Product/1  "<azsign>"
  Parameters/1 -> Bus Selector/1, Bus Assignment/1
  Bus Assignment/1 -> Propeller Rotation Dynamics/1
  For Iterator/1 -> Selector3/2, Selector2/2, Selector1/2, Assignment1/2, Selector7/2
  Orientation/1 -> Propeller Rotation Dynamics/2
  omega_B_E_B/1 -> Propeller Rotation Dynamics/5
  torque_prop/1 -> Selector1/1
  Selector1/1 -> Propeller Rotation Dynamics/3
  omega_dot_B_E_B/1 -> Propeller Rotation Dynamics/6
  Selector2/1 -> Propeller Rotation Dynamics/7
  Assignment1/1 -> omega_dot_motors/1
  Propeller Rotation Dynamics/1 -> Assignment1/1

== system UAVdesign_net/Vehicle Models/Quad-Rotor Model (Momentum)/Fuselage ==
  Parameters : Inport
  Environment : Inport  Port=2
  R_IELA_B_B : Inport  Port=3  PortDimensions=3
  T_IERA_IELA : Inport  Port=4  PortDimensions=[3 3]
  V_B_E_B : Inport  Port=5  PortDimensions=3
  omega_B_E_B : Inport  Port=6  PortDimensions=3
  V_W : Inport  Port=7  PortDimensions=3
  omega_W : Inport  Port=8  PortDimensions=3
  CG to IELA : Subsystem
      mask Display:
      | port_label('input', 1, 'R_{IELA-B|B}', 'texmode', 'on')
      | port_label('input', 2, 'V_{B-E|B}', 'texmode', 'on')
      | port_label('input', 3, '\omega_{B-E|B}', 'texmode', 'on')
      | port_label('output', 1, 'V_{IELA-E|IELA}', 'texmode', 'on')
      | port_label('output', 2, '\omega_{IELA-E|IELA}', 'texmode', 'on')
  Fuselage Model (IERA) : Subsystem
      mask Display:
      | port_label('input', 1, 'Parameters', 'texmode', 'on')
      | port_label('input', 2, 'Environment', 'texmode', 'on')
      | port_label('input', 3, 'V_{A}', 'texmode', 'on')
      | port_label('input', 4, '\omega_{A}', 'texmode', 'on')
      | port_label('input', 5, 'V_{W}', 'texmode', 'on')
      | port_label('input', 6, '\omega_{W}', 'texmode', 'on')
      | 
      | port_label('output', 1, 'FM_{I}', 'texmode', 'on')
      | port_label('output', 2, 'FM_{A}', 'texmode', 'on')
      | port_label('output', 3, 'd_{k}', 'texmode', 'on')
  IELA to CG : Subsystem
      mask Display:
      | port_label('input', 1, 'R_{IELA-B|B}', 'texmode', 'on')
      | port_label('input', 2, 'FM_{IELA}', 'texmode', 'on')
      | port_label('output', 1, 'FM_{B}', 'texmode', 'on')
  IELA to IERA : Subsystem
      mask Display:
      | port_label('input', 1, 'T_{IERA-IELA}', 'texmode', 'on')
      | port_label('input', 2, 'V_{A|IELA}', 'texmode', 'on')
      | port_label('input', 3, '\omega_{A|IELA}', 'texmode', 'on')
      | port_label('input', 4, 'V_{W|IELA}', 'texmode', 'on')
      | port_label('input', 5, '\omega_{W|IELA}', 'texmode', 'on')
      | 
      | port_label('output', 1, 'V_{A|IERA}', 'texmode', 'on')
      | port_label('output', 2, '\omega_{A|IERA}', 'texmode', 'on')
      | port_label('output', 3, 'V_{W|IERA}', 'texmode', 'on')
      | port_label('output', 4, '\omega_{W|IERA}', 'texmode', 'on')
  IERA to IELA : Subsystem
      mask Display:
      | port_label('input', 1, 'T_{IELA-IERA}', 'texmode', 'on')
      | port_label('input', 2, 'FM_{I|IERA}', 'texmode', 'on')
      | port_label('input', 3, 'FM_{A|IERA}', 'texmode', 'on')
      | port_label('input', 4, 'd_{IERA}', 'texmode', 'on')
      | port_label('output', 1, 'FM_{I|IELA}', 'texmode', 'on')
      | port_label('output', 2, 'FM_{A|IELA}', 'texmode', 'on')
      | port_label('output', 3, 'd_{IELA}', 'texmode', 'on')
  Sum : Sum  Inputs=++|
  Sum3 : Sum  Inputs=|+-
  Sum4 : Sum  Inputs=|+-
  Transpose : Subsystem
      mask Display: disp('A^T', 'texmode', 'on')
  Vector Concatenate : Concatenate  Mode=Vector
  FM_B : Outport  PortDimensions=6
  FM_IELA : Outport  Port=2  PortDimensions=6
  d (k) : Outport  Port=3  PortDimensions=3
  V_om_A : Outport  Port=4  PortDimensions=6
  wires:
  Vector Concatenate/1 -> V_om_A/1
  omega_W/1 -> IELA to IERA/5(omega_W_IELA), Sum4/2
  V_W/1 -> IELA to IERA/4(V_W_IELA), Sum3/2
  Sum4/1 -> Vector Concatenate/2, IELA to IERA/3(omega_A_IELA)
  CG to IELA/2(omega_IELA-E|IELA) -> Sum4/1
  Sum3/1 -> Vector Concatenate/1, IELA to IERA/2(V_A_IELA)
  CG to IELA/1(V_IELA-E|IELA) -> Sum3/1
  R_IELA_B_B/1 -> IELA to CG/1(R_IELA_B_B), CG to IELA/1(R_IELA-B|B)
  IERA to IELA/3(d_IELA) -> d (k)/1
  IELA to CG/1(FM_B) -> FM_B/1
  Transpose/1(Out) -> IERA to IELA/1(T_IELA_IERA)
  V_B_E_B/1 -> CG to IELA/2(V_B-E|B)
  T_IERA_IELA/1 -> Transpose/1(In), IELA to IERA/1(T_IERA_IELA)
  Environment/1 -> Fuselage Model (IERA)/2(Environment)
  Parameters/1 -> Fuselage Model (IERA)/1(Parameters)
  Fuselage Model (IERA)/3(d (k)) -> IERA to IELA/4(d_IERA)
  IERA to IELA/2(FM_A_IELA) -> Sum/2
  IELA to IERA/4(omega_W_IERA) -> Fuselage Model (IERA)/6(omega_W)
  IELA to IERA/3(V_W_IERA) -> Fuselage Model (IERA)/5(V_W)
  IELA to IERA/2(omega_A_IERA) -> Fuselage Model (IERA)/4(omega_A)
  IELA to IERA/1(V_A_IERA) -> Fuselage Model (IERA)/3(V_A)
  omega_B_E_B/1 -> CG to IELA/3(omega_B_E|B)
  Fuselage Model (IERA)/1(FM_I) -> IERA to IELA/2(FM_I_IERA)
  Fuselage Model (IERA)/2(FM_A) -> IERA to IELA/3(FM_A_IERA)
  Sum/1 -> FM_IELA/1, IELA to CG/2(FM_IELA)
  IERA to IELA/1(FM_I_IELA) -> Sum/1

== system UAVdesign_net/Vehicle Models/Quad-Rotor Model (Momentum)/RA to IELA CG computation ==
  Geometry : Inport
  Body Coordinates Computation : Subsystem  TreatAsAtomicUnit=on
  Divide : Product  Inputs=*/
  GC Computation : Subsystem  TreatAsAtomicUnit=on
  Selector : Selector  InputPortWidth=18  IndexOptions=Index vector (dialog)  Indices=[16:18]  OutputSizes=1
  Selector1 : Selector  InputPortWidth=18  IndexOptions=Index vector (dialog)  Indices=[4:15]  OutputSizes=1
  Selector2 : Selector  NumberOfDimensions=2  InputPortWidth=18  IndexOptions=Index vector (dialog),Index vector (dialog)  Indices=[1:3],[16:18]  OutputSizes=1,1
  Selector3 : Selector  NumberOfDimensions=2  InputPortWidth=18  IndexOptions=Index vector (dialog),Index vector (dialog)  Indices=[1:3],[4:6]  OutputSizes=1,1
  mass : Outport
  In_B : Outport  Port=2
  FUSE_R_IELA_B_B : Outport  Port=3
  FUSE_T_IERA_IELA : Outport  Port=4
  ROT_R_IELA_B_B : Outport  Port=5
  ROT_T_IERA_IELA : Outport  Port=6
  wires:
  Geometry/1 -> Body Coordinates Computation/1(Geometry), GC Computation/1(Geometry)
  Body Coordinates Computation/3(Inb) -> In_B/1
  GC Computation/2(mass) -> mass/1, Divide/2
  Selector/1 -> FUSE_R_IELA_B_B/1
  Selector1/1 -> ROT_R_IELA_B_B/1
  Body Coordinates Computation/1(R_IERA_B_B) -> Selector/1, Selector1/1
  Selector2/1 -> FUSE_T_IERA_IELA/1
  Body Coordinates Computation/2(T_IERA_IELA) -> Selector2/1, Selector3/1
  Selector3/1 -> ROT_T_IERA_IELA/1
  GC Computation/1(R_CG_RA_RA_m) -> Divide/1
  Divide/1 -> Body Coordinates Computation/2(R_CG_RA_RA)

== system UAVdesign_net/Vehicle Models/Quad-Rotor Model (Momentum)/Wash Coupling ==
  ParametersBus : Inport
  GeometryBus : Inport  Port=2
  d_vector : Inport  Port=3
  Wind : Inport  Port=4
  Bus Selector : BusSelector  OutputSignals=ROT.radius
  Bus Selector1 : BusSelector  OutputSignals=ROT1.R_IERA_RA_RA,ROT2.R_IERA_RA_RA,ROT3.R_IERA_RA_RA,ROT4.R_IERA_RA_RA,FUSE.R_IERA_RA_RA
  Vector Concatenate1 : Concatenate  NumInputs=5  Mode=Vector
  Wash Coupling : Stateflow chart  TreatAsAtomicUnit=on
  V_W_omega_W_vector : Outport
  wires:
  d_vector/1 -> Wash Coupling/1(d)
  Wash Coupling/1(vw_omw) -> V_W_omega_W_vector/1
  ParametersBus/1 -> Bus Selector/1
  Bus Selector/1 -> Wash Coupling/3(ROT_radius)  "<radius>"
  GeometryBus/1 -> Bus Selector1/1
  Vector Concatenate1/1 -> Wash Coupling/2(R)
  Bus Selector1/1 -> Vector Concatenate1/1  "<R_IERA_RA_RA>"
  Bus Selector1/2 -> Vector Concatenate1/2  "<R_IERA_RA_RA>"
  Bus Selector1/3 -> Vector Concatenate1/3  "<R_IERA_RA_RA>"
  Bus Selector1/4 -> Vector Concatenate1/4  "<R_IERA_RA_RA>"
  Bus Selector1/5 -> Vector Concatenate1/5  "<R_IERA_RA_RA>"
  Wind/1 -> Wash Coupling/4(wind)

== system UAVdesign_net/Vehicle Models/QuadRotor Parameters/Fuse Parameters ==
  In : Inport
  Bus Creator : BusCreator  Inputs=7  OutDataTypeStr=Bus: FuselageParameters  NonVirtualBus=on
  Demux : Demux  Outputs=17
  Vector Concatenate{,1..4} (5 alike) : Concatenate  NumInputs=3  Mode=Vector
  Parameters : Outport  OutDataTypeStr=Bus: FuselageParameters
  wires:
  Vector Concatenate4/1 -> Bus Creator/7  "cn"
  Vector Concatenate3/1 -> Bus Creator/6  "cm"
  Demux/17 -> Vector Concatenate4/3
  Demux/16 -> Vector Concatenate4/2
  Demux/15 -> Vector Concatenate4/1
  Demux/14 -> Vector Concatenate3/3
  Demux/13 -> Vector Concatenate3/2
  Demux/12 -> Vector Concatenate3/1
  Vector Concatenate2/1 -> Bus Creator/5  "cz"
  Demux/11 -> Vector Concatenate2/3
  Demux/10 -> Vector Concatenate2/2
  Demux/9 -> Vector Concatenate2/1
  Vector Concatenate1/1 -> Bus Creator/4  "cy"
  Demux/8 -> Vector Concatenate1/3
  Demux/7 -> Vector Concatenate1/2
  Demux/6 -> Vector Concatenate1/1
  Vector Concatenate/1 -> Bus Creator/3  "cx"
  Demux/5 -> Vector Concatenate/3
  Demux/4 -> Vector Concatenate/2
  Demux/3 -> Vector Concatenate/1
  Demux/2 -> Bus Creator/2  "clen"
  In/1 -> Demux/1
  Bus Creator/1 -> Parameters/1
  Demux/1 -> Bus Creator/1  "carea"

== system UAVdesign_net/Vehicle Models/QuadRotor Parameters/Motor Parameters ==
  In : Inport
  Bus Creator1 : BusCreator  Inputs=7  NonVirtualBus=on
  Data Type Conversion2 : DataTypeConversion  OutDataTypeStr=uint32  RndMeth=Nearest
  Demux1 : Demux  Outputs=7
  Parameters : Outport
  wires:
  Demux1/7 -> Bus Creator1/7  "Ngear"
  Demux1/6 -> Bus Creator1/6  "In"
  Data Type Conversion2/1 -> Bus Creator1/5  "poles"
  Demux1/5 -> Data Type Conversion2/1
  Demux1/4 -> Bus Creator1/4  "Kt"
  Demux1/3 -> Bus Creator1/3  "Kv"
  Demux1/2 -> Bus Creator1/2  "L"
  Demux1/1 -> Bus Creator1/1  "R"
  Bus Creator1/1 -> Parameters/1
  In/1 -> Demux1/1

== system UAVdesign_net/Vehicle Models/QuadRotor Parameters/Rotor Parameters ==
  In : Inport
  Bus Creator1 : BusCreator  Inputs=14  NonVirtualBus=on
  Data Type Conversion1 : DataTypeConversion  OutDataTypeStr=uint32  RndMeth=Nearest
  Data Type Conversion2 : DataTypeConversion  OutDataTypeStr=uint32  RndMeth=Nearest
  Demux1 : Demux  Outputs=16
  Gain1 : Gain  Gain=pi/180
  Gain3 : Gain  Gain=pi/180
  Vector Concatenate : Concatenate  NumInputs=3  Mode=Vector
  Parameters : Outport
  wires:
  Data Type Conversion2/1 -> Bus Creator1/14  "flags"
  Demux1/16 -> Data Type Conversion2/1
  Gain3/1 -> Bus Creator1/10  "twist"
  Vector Concatenate/1 -> Bus Creator1/2  "del0_2"
  Gain1/1 -> Bus Creator1/9  "theta"
  Demux1/11 -> Gain1/1  "theta"
  Demux1/10 -> Bus Creator1/8  "btq"
  Demux1/12 -> Gain3/1
  Demux1/8 -> Bus Creator1/6  "btmin"
  Demux1/7 -> Bus Creator1/5  "chord"
  Demux1/6 -> Bus Creator1/4  "radius"
  Demux1/5 -> Data Type Conversion1/1
  Data Type Conversion1/1 -> Bus Creator1/3  "nb"
  In/1 -> Demux1/1
  Demux1/2 -> Vector Concatenate/1
  Demux1/3 -> Vector Concatenate/2
  Demux1/4 -> Vector Concatenate/3
  Bus Creator1/1 -> Parameters/1
  Demux1/1 -> Bus Creator1/1  "a0"
  Demux1/9 -> Bus Creator1/7  "btmax"
  Demux1/13 -> Bus Creator1/11  "iflap"
  Demux1/14 -> Bus Creator1/12  "mbar"
  Demux1/15 -> Bus Creator1/13  "azsign"

== system UAVdesign_net/Subsystem Models/Fin/Fin Model (IERA)/Fin ==
  Parameters : Inport  OutDataTypeStr=Bus: FinParameters
  Environment : Inport  Port=2  OutDataTypeStr=Bus: Environment
  V_A : Inport  Port=3
  omega_A : Inport  Port=4
  T_WRA_MAC : Inport  Port=5
  T_MAC_WRA : Inport  Port=6
  Bus Selector : BusSelector  OutputSignals=taper,span,sweep,dihedral
  Fin Forces and Moments : Subsystem
      mask Display:
      | port_label('input', 1, 'Parameters', 'texmode', 'on')
      | port_label('input', 2, 'Environment', 'texmode', 'on')
      | port_label('input', 3, 'V_{A|WRA}', 'texmode', 'on')
      | port_label('input', 4, '\omega_{A|WRA}', 'texmode', 'on')
      | 
      | port_label('output', 1, 'FM_{A}', 'texmode', 'on')
  IERA to MAC : Subsystem
      mask Display:
      | port_label('input', 1, 'R_{MAC-IERA|IERA}', 'texmode', 'on')
      | port_label('input', 2, 'V_{A|IERA}', 'texmode', 'on')
      | port_label('input', 3, '\omega_{A|IERA}', 'texmode', 'on')
      | port_label('output', 1, 'V_{A|MAC}', 'texmode', 'on')
      | port_label('output', 2, '\omega_{A|MAC}', 'texmode', 'on')
  MAC to IERA : Subsystem
      mask Display:
      | port_label('input', 1, 'R_{MAC-IERA|IERA}', 'texmode', 'on')
      | port_label('input', 2, 'FM_{MAC}', 'texmode', 'on')
      | port_label('output', 1, 'FM_{IERA}', 'texmode', 'on')
  MAC to WRA (Half Wing) : Subsystem
      mask Display:
      | port_label('input', 1, 'T_{WRA-MAC}', 'texmode', 'on')
      | port_label('input', 2, 'V_{A|MAC}', 'texmode', 'on')
      | port_label('input', 3, '\omega_{A|MAC}', 'texmode', 'on')
      | 
      | port_label('output', 1, 'V_{A|WRA}', 'texmode', 'on')
      | port_label('output', 2, '\omega_{A|WRA}', 'texmode', 'on')
  Mux1 : Mux  Inputs=3
  Mux2 : Mux  Inputs=2
  Mux3 : Mux  Inputs=3
  WRA to MAC : Subsystem
      mask Display:
      | port_label('input', 1, 'T_{MAC-WRA}', 'texmode', 'on')
      | port_label('input', 2, 'FM_{A|WRA}', 'texmode', 'on')
      | 
      | port_label('output', 1, 'FM_{A|MAC}', 'texmode', 'on')
  smac : Fcn  Expr=2 * u(2) * (2 * u(1) + 1) / 6 / (u(1) + 1)
  xmac : Fcn  Expr=-sin(u(2)) * cos(-u(3)) * u(1)
  ymac : Fcn  Expr=cos(u(2)) * cos(-u(3)) * u(1)
  zmac : Fcn  Expr=sin(-u(3)) * u(1)
  FM_A : Outport
  wires:
  Fin Forces and Moments/1(FM_A) -> WRA to MAC/2(FM_A_WM)
  IERA to MAC/1(V_A|MAC) -> MAC to WRA (Half Wing)/2(V_A_MAC)
  IERA to MAC/2(omega_A|MAC) -> MAC to WRA (Half Wing)/3(omega_A_MAC)
  zmac/1 -> Mux3/3
  ymac/1 -> Mux3/2
  xmac/1 -> Mux3/1
  Mux3/1 -> IERA to MAC/1(R_xW-IERA|IERA), MAC to IERA/1(R_MAC_IERA_IERA)
  MAC to WRA (Half Wing)/1(V_A_WRA) -> Fin Forces and Moments/3(V_A)
  MAC to WRA (Half Wing)/2(omega_A_WRA) -> Fin Forces and Moments/4(omega_A)
  Parameters/1 -> Fin Forces and Moments/1(Parameters), Bus Selector/1
  T_WRA_MAC/1 -> MAC to WRA (Half Wing)/1(T_WRA_MAC)
  T_MAC_WRA/1 -> WRA to MAC/1(T_IERA_WM)
  V_A/1 -> IERA to MAC/2(V_A|IERA)
  omega_A/1 -> IERA to MAC/3(omega_A|IERA)
  Mux1/1 -> ymac/1, xmac/1, zmac/1
  smac/1 -> Mux1/1
  Environment/1 -> Fin Forces and Moments/2(Environment)
  Bus Selector/1 -> Mux2/1  "<taper>"
  Bus Selector/2 -> Mux2/2  "<span>"
  Mux2/1 -> smac/1
  Bus Selector/3 -> Mux1/2  "<sweep>"
  Bus Selector/4 -> Mux1/3  "<dihedral>"
  WRA to MAC/1(FM_A_IERA) -> MAC to IERA/2(FM_MAC)
  MAC to IERA/1(FM_IERA) -> FM_A/1

== system UAVdesign_net/Subsystem Models/Fin/Fin Model (IERA)/Fin Self-Influence ==
  Parameters : Inport  OutDataTypeStr=Bus: FinParameters
  Environment : Inport  Port=2  OutDataTypeStr=Bus: Environment
  V_A : Inport  Port=3
  omega_A : Inport  Port=4
  FM_A : Inport  Port=5
  Fin Wash Self-Influence (IERA) : Stateflow chart  TreatAsAtomicUnit=on
  d (k) : Outport
  wires:
  FM_A/1 -> Fin Wash Self-Influence (IERA)/5(FM_A)
  omega_A/1 -> Fin Wash Self-Influence (IERA)/4(oma)
  V_A/1 -> Fin Wash Self-Influence (IERA)/3(va)
  Environment/1 -> Fin Wash Self-Influence (IERA)/2(Environment)
  Fin Wash Self-Influence (IERA)/1(d) -> d (k)/1
  Parameters/1 -> Fin Wash Self-Influence (IERA)/1(Parameters)

== system UAVdesign_net/Subsystem Models/Fin/Fin Model (IERA)/Transpose ==
  In : Inport
  Permute Dimensions : PermuteDimensions
  Out : Outport
  wires:
  Permute Dimensions/1 -> Out/1
  In/1 -> Permute Dimensions/1

== system UAVdesign_net/Subsystem Models/Fuselage/Fuselage Model (IERA)/Fuselage Forces and Moments ==
  Parameters : Inport  OutDataTypeStr=Bus: FuselageParameters
  Environment : Inport  Port=2  OutDataTypeStr=Bus: Environment
  V_A : Inport  Port=3
  omega_A : Inport  Port=4
  Fuselage Forces and Moments : Stateflow chart  TreatAsAtomicUnit=on
  FM_A : Outport
  wires:
  Fuselage Forces and Moments/1(FM_A) -> FM_A/1
  omega_A/1 -> Fuselage Forces and Moments/4(oma)
  V_A/1 -> Fuselage Forces and Moments/3(va)
  Environment/1 -> Fuselage Forces and Moments/2(Environment)
  Parameters/1 -> Fuselage Forces and Moments/1(Parameters)

== system UAVdesign_net/Subsystem Models/Fuselage/Fuselage Model (IERA)/Fuselage Self-Influence ==
  Parameters : Inport  OutDataTypeStr=Bus: FuselageParameters
  Environment : Inport  Port=2  OutDataTypeStr=Bus: Environment
  V_A : Inport  Port=3
  omega_A : Inport  Port=4
  FM_A : Inport  Port=5
  Fuselage Wash Self-Influence : Stateflow chart  TreatAsAtomicUnit=on
  d (k) : Outport
  wires:
  FM_A/1 -> Fuselage Wash Self-Influence/5(FM_A)
  omega_A/1 -> Fuselage Wash Self-Influence/4(oma)
  V_A/1 -> Fuselage Wash Self-Influence/3(va)
  Environment/1 -> Fuselage Wash Self-Influence/2(Environment)
  Fuselage Wash Self-Influence/1(d) -> d (k)/1
  Parameters/1 -> Fuselage Wash Self-Influence/1(Parameters)

== system UAVdesign_net/Subsystem Models/Helicopter Rotor/Rotor Model (IERA)/IERA to WM ==
  T_WM_IERA : Inport
  V_I_IERA : Inport  Port=2
  omega_I_IERA : Inport  Port=3
  V_dot_I_IERA : Inport  Port=4
  omega_dot_I_IERA : Inport  Port=5
  V_A_IERA : Inport  Port=6
  omega_A_IERA : Inport  Port=7
  controls_IERA : Inport  Port=8
  flap_IERA : Inport  Port=9
  1D : Reshape
  Constant : Constant  Value=0
  Constant1 : Constant  Value=0
  Demux : Demux  Outputs=6
  Demux{1..4} (4 alike) : Demux  Outputs=3
  Mux{,1..3} (4 alike) : Mux  Inputs=3
  Product : Product  Multiplication=Matrix(*)  RndMeth=Zero
  Product1 : Product  Multiplication=Matrix(*)  RndMeth=Zero
  Product2 : Product  Multiplication=Matrix(*)  RndMeth=Zero
  Terminator : Terminator
  Terminator1 : Terminator
  Vector Concatenate : Concatenate  NumInputs=6  Mode=Multidimensional array  ConcatenateDimension=2
  V_I_WM : Outport
  omega_I_WM : Outport  Port=2
  V_dot_I_WM : Outport  Port=3
  omega_dot_I_WM : Outport  Port=4
  V_A_WM : Outport  Port=5
  omega_A_WM : Outport  Port=6
  controls_WM : Outport  Port=7
  flap_WM : Outport  Port=8
  wires:
  Demux4/3 -> Terminator1/1
  Demux4/2 -> Mux2/2
  Demux4/1 -> Mux2/3
  Product2/1 -> Demux4/1
  Mux3/1 -> Product2/2
  Constant1/1 -> Mux3/3
  Demux3/3 -> Mux3/1  "b1"
  Demux3/2 -> Mux3/2  "a1"
  Demux3/1 -> Mux2/1  "beta"
  Mux2/1 -> flap_WM/1
  flap_IERA/1 -> Demux3/1
  Demux2/3 -> Terminator/1
  Demux2/2 -> Mux/2
  Demux2/1 -> Mux/3
  Product1/1 -> Demux2/1
  Constant/1 -> Mux1/3
  Demux1/2 -> Mux1/2  "A1"
  Demux1/3 -> Mux1/1  "B1"
  Mux1/1 -> Product1/2
  Demux1/1 -> Mux/1  "collective"
  controls_IERA/1 -> Demux1/1
  Mux/1 -> controls_WM/1
  T_WM_IERA/1 -> Product2/1, Product1/1, Product/1
  V_I_IERA/1 -> Vector Concatenate/1
  omega_I_IERA/1 -> Vector Concatenate/2
  V_dot_I_IERA/1 -> Vector Concatenate/3
  omega_dot_I_IERA/1 -> Vector Concatenate/4
  V_A_IERA/1 -> Vector Concatenate/5
  omega_A_IERA/1 -> Vector Concatenate/6
  Vector Concatenate/1 -> Product/2
  Product/1 -> 1D/1
  1D/1 -> Demux/1
  Demux/1 -> V_I_WM/1
  Demux/2 -> omega_I_WM/1
  Demux/3 -> V_dot_I_WM/1
  Demux/4 -> omega_dot_I_WM/1
  Demux/5 -> V_A_WM/1
  Demux/6 -> omega_A_WM/1
